simulink model "test_vehicle_model"  (R2016b)
settings: Solver=VariableStepAuto  StartTime=t_start  StopTime=t_stop  RelTol=1e-9  EnableMultiTasking=on
values from neighbouring files (symbols this model uses):
  a = 3.75    [test_vehicle.m]    (also in test_vehicle_model.m = 3.5)
  B = 5    [test_vehicle.m]    (also in test_vehicle_model.m)
  b = L - a    (= 3.25)    [test_vehicle.m]    (also in test_vehicle_model.m = 3.5)
  disturb_time = 5    [test_vehicle.m]
  disturb_val = 20    [test_vehicle.m]
  gear_ratio = 1/4.1    (= 0.243902439024)    [test_vehicle.m]    (also in test_vehicle_model.m = 1)
  I = 210000/(12^2)    (= 1458.33333333)    [test_vehicle.m]    (also in test_vehicle_model.m = 217852)
  input = [5000 50]    [test_vehicle.m]
  k_motor = 167    [test_vehicle.m]    (also in test_vehicle_model.m = 1)
  Ka = m*.15*180/(2*pi)    (= 40.0358707778)    [test_vehicle.m]    (also in test_vehicle_model.m = 0.5)
  Kx = m*.15*180/(2*pi)    (= 40.0358707778)    [test_vehicle.m]    (also in test_vehicle_model.m = 0.5)
  m = 300/32.2    (= 9.31677018634)    [test_vehicle.m]    (also in test_vehicle_model.m = 150)
  R = 4/12    (= 0.333333333333)    [test_vehicle.m]
  speed_D = 0    [test_vehicle.m]
  speed_I = 0    [test_vehicle.m]
  speed_N = 100    [test_vehicle.m]
  speed_P = 100    [test_vehicle.m]
  speed_sp = 30    [test_vehicle.m]
  steer_D = 0.1    [test_vehicle.m]
  steer_I = 0    [test_vehicle.m]
  steer_N = 1000    [test_vehicle.m]
  steer_P = 10    [test_vehicle.m]
  t_motor = 0.025    [test_vehicle.m]    (also in test_vehicle_model.m = 1)
  u_start = 0.01    [test_vehicle.m]
libraries: simulink x2
settings Model: Creator=jbarr  LastModifiedBy=john
settings SolverCC: ZeroCrossAlgorithm=Adaptive
settings OptimizationCC: LifeSpan=1
settings DebuggingCC: SFExecutionAtInitializationDiag=none

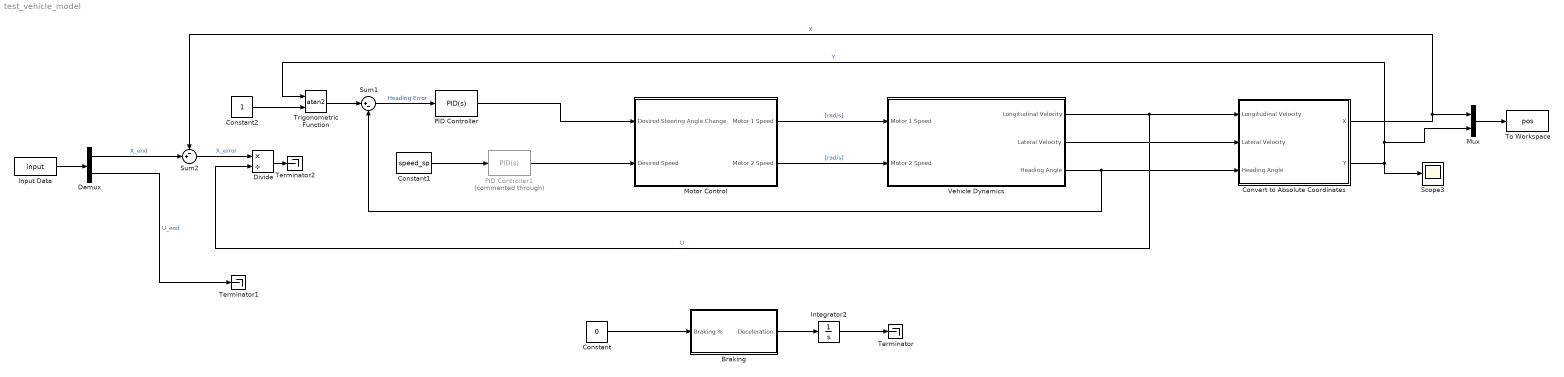
== system test_vehicle_model ==
  "Braking " : Subsystem
  Constant : Constant  Value=0
  Constant1 : Constant  Value=speed_sp
  Constant2 : Constant
  Convert to Absolute Coordinates : Subsystem
  Demux : Demux  Outputs=2
  Divide : Product  Inputs=*/
  Input Data : Constant  Value=input
  Integrator2 : Integrator  InitialCondition=0.001
  "Motor Control " : Subsystem
  Mux : Mux  Inputs=2
  PID Controller : simulink/Continuous/PID Controller  Controller=PID  TimeDomain=Continuous-time  SampleTime=-1  IntegratorMethod=Forward Euler  FilterMethod=Forward Euler  Form=Ideal  UseFilter=on  ControllerParametersSource=internal  P=steer_P  I=steer_I  D=steer_D  N=steer_N  InitialConditionSource=internal  InitialConditionForIntegrator=0  InitialConditionForFilter=0  ExternalReset=none  LimitOutput=off  UpperSaturationLimit=100  LowerSaturationLimit=0  LinearizeAsGain=on  AntiWindupMode=none  Kb=1  TrackingMode=off  Kt=1  PParamMin=[]  PParamMax=[]  IParamMin=[]  IParamMax=[]  DParamMin=[]  DParamMax=[]  NParamMin=[]  NParamMax=[]  KbParamMin=[]  KbParamMax=[]  KtParamMin=[]  KtParamMax=[]  POutMin=[]  POutMax=[]  IOutMin=[]  IOutMax=[]  DOutMin=[]  DOutMax=[]  NOutMin=[]  NOutMax=[]  KbOutMin=[]  KbOutMax=[]  KtOutMin=[]  KtOutMax=[]  IntegratorOutMin=[]  IntegratorOutMax=[]  FilterOutMin=[]  FilterOutMax=[]  SumOutMin=[]  SumOutMax=[]  SumI1OutMin=[]  SumI1OutMax=[]  SumI2OutMin=[]  SumI2OutMax=[]  SumI3OutMin=[]  SumI3OutMax=[]  SumDOutMin=[]  SumDOutMax=[]  SaturationOutMin=[]  SaturationOutMax=[]  IntegratorContinuousStateAttributes=''  IntegratorStateMustResolveToSignalObject=off  IntegratorRTWStateStorageClass=Auto  FilterContinuousStateAttributes=''  FilterStateMustResolveToSignalObject=off  FilterRTWStateStorageClass=Auto  DifferentiatorICPrevScaledInput=0  DifferentiatorOutMin=[]  DifferentiatorOutMax=[]
  PID Controller1 : simulink/Continuous/PID Controller  Commented=through  Controller=PID  TimeDomain=Continuous-time  SampleTime=-1  IntegratorMethod=Forward Euler  FilterMethod=Forward Euler  Form=Ideal  UseFilter=on  ControllerParametersSource=internal  P=speed_P  I=speed_I  D=speed_D  N=speed_N  InitialConditionSource=internal  InitialConditionForIntegrator=0  InitialConditionForFilter=0  ExternalReset=none  LimitOutput=off  UpperSaturationLimit=100  LowerSaturationLimit=0  LinearizeAsGain=on  AntiWindupMode=none  Kb=1  TrackingMode=off  Kt=1  PParamMin=[]  PParamMax=[]  IParamMin=[]  IParamMax=[]  DParamMin=[]  DParamMax=[]  NParamMin=[]  NParamMax=[]  KbParamMin=[]  KbParamMax=[]  KtParamMin=[]  KtParamMax=[]  POutMin=[]  POutMax=[]  IOutMin=[]  IOutMax=[]  DOutMin=[]  DOutMax=[]  NOutMin=[]  NOutMax=[]  KbOutMin=[]  KbOutMax=[]  KtOutMin=[]  KtOutMax=[]  IntegratorOutMin=[]  IntegratorOutMax=[]  FilterOutMin=[]  FilterOutMax=[]  SumOutMin=[]  SumOutMax=[]  SumI1OutMin=[]  SumI1OutMax=[]  SumI2OutMin=[]  SumI2OutMax=[]  SumI3OutMin=[]  SumI3OutMax=[]  SumDOutMin=[]  SumDOutMax=[]  SaturationOutMin=[]  SaturationOutMax=[]  IntegratorContinuousStateAttributes=''  IntegratorStateMustResolveToSignalObject=off  IntegratorRTWStateStorageClass=Auto  FilterContinuousStateAttributes=''  FilterStateMustResolveToSignalObject=off  FilterRTWStateStorageClass=Auto  DifferentiatorICPrevScaledInput=0  DifferentiatorOutMin=[]  DifferentiatorOutMax=[]
  Scope3 : Scope
  Sum1 : Sum  Inputs=|+-
  Sum2 : Sum  Inputs=-+|
  Terminator : Terminator
  Terminator1 : Terminator
  Terminator2 : Terminator
  To Workspace : ToWorkspace  VariableName=pos  SampleTime=-1
  Trigonometric Function : Trigonometry  Operator=atan2
  Vehicle Dynamics : Subsystem
  wires:
  "Motor Control "/1(Motor 1 Speed) -> Vehicle Dynamics/1(Motor 1 Speed)  "[rad/s]"
  Mux/1 -> To Workspace/1
  Convert to Absolute Coordinates/2(Y) -> Scope3/1, Trigonometric Function/1, Mux/2  "Y"
  Convert to Absolute Coordinates/1(X) -> Sum2/1, Mux/1  "X"
  "Braking "/1(Deceleration) -> Integrator2/1
  Vehicle Dynamics/1(Longitudinal Velocity) -> Divide/2, Convert to Absolute Coordinates/1(Longitudinal Velocity)  "U"
  Constant/1 -> "Braking "/1(Braking %)
  Sum1/1 -> PID Controller/1  "Heading Error"
  "Motor Control "/2(Motor 2 Speed) -> Vehicle Dynamics/2(Motor 2 Speed)  "[rad/s]"
  PID Controller/1 -> "Motor Control "/1(Desired Steering Angle Change)
  PID Controller1/1 -> "Motor Control "/2(Desired Speed)
  Integrator2/1 -> Terminator/1
  Vehicle Dynamics/2(Lateral Velocity) -> Convert to Absolute Coordinates/2(Lateral Velocity)
  Input Data/1 -> Demux/1
  Demux/1 -> Sum2/2  "X_end"
  Sum2/1 -> Divide/1  "X_error"
  Demux/2 -> Terminator1/1  "U_end"
  Trigonometric Function/1 -> Sum1/1
  Constant1/1 -> PID Controller1/1
  Divide/1 -> Terminator2/1
  Vehicle Dynamics/3(Heading Angle) -> Sum1/2, Convert to Absolute Coordinates/3(Heading Angle)
  Constant2/1 -> Trigonometric Function/2

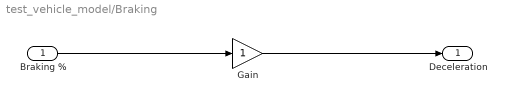
== system test_vehicle_model/Braking  ==
  Braking % : Inport
  Gain : Gain
  Deceleration : Outport
  wires:
  Gain/1 -> Deceleration/1
  Braking %/1 -> Gain/1

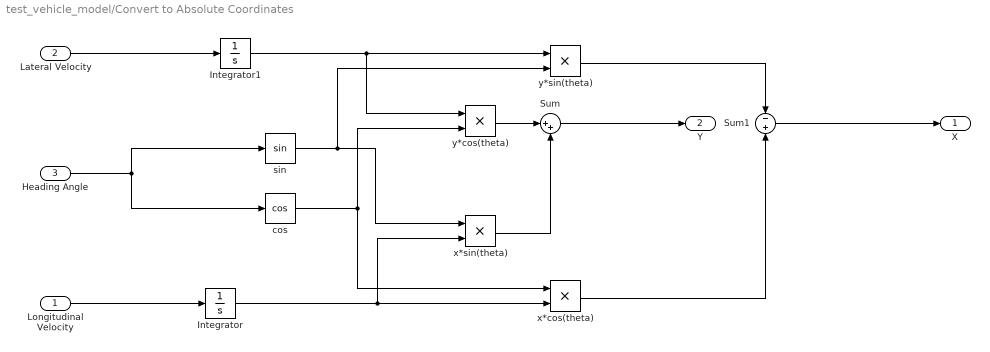
== system test_vehicle_model/Convert to Absolute Coordinates ==
  Longitudinal Velocity : Inport
  Lateral Velocity : Inport  Port=2
  Heading Angle : Inport  Port=3
  Integrator : Integrator  InitialCondition=0.001
  Integrator1 : Integrator
  Sum : Sum  Inputs=|++
  Sum1 : Sum  Inputs=-+
  cos : Trigonometry  Operator=cos
  sin : Trigonometry
  x*cos(theta) : Product
  x*sin(theta) : Product
  y*cos(theta) : Product
  y*sin(theta) : Product
  X : Outport
  Y : Outport  Port=2
  wires:
  Longitudinal Velocity/1 -> Integrator/1
  cos/1 -> y*cos(theta)/2, x*cos(theta)/1
  sin/1 -> x*sin(theta)/1, y*sin(theta)/2
  x*cos(theta)/1 -> Sum1/2
  x*sin(theta)/1 -> Sum/2
  y*cos(theta)/1 -> Sum/1
  y*sin(theta)/1 -> Sum1/1
  Integrator1/1 -> y*cos(theta)/1, y*sin(theta)/1
  Integrator/1 -> x*sin(theta)/2, x*cos(theta)/2
  Heading Angle/1 -> sin/1, cos/1
  Sum1/1 -> X/1
  Lateral Velocity/1 -> Integrator1/1
  Sum/1 -> Y/1

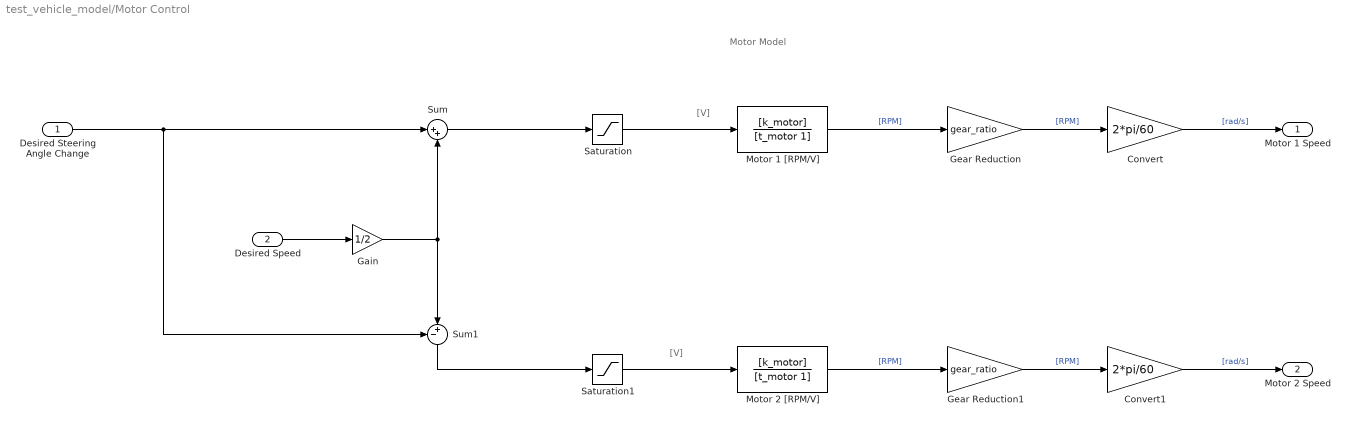
== system test_vehicle_model/Motor Control  ==
  note: [V]
  note: Motor Model
  note: [V]
  Desired Steering Angle Change : Inport
  Desired Speed : Inport  Port=2
  Convert : Gain  Gain=2*pi/60
  Convert1 : Gain  Gain=2*pi/60
  Gain : Gain  Gain=1/2
  Gear Reduction : Gain  Gain=gear_ratio
  Gear Reduction1 : Gain  Gain=gear_ratio
  "Motor 1 [RPM/V] " : TransferFcn  Numerator=[k_motor]  Denominator=[t_motor 1]
  Motor 2 [RPM/V] : TransferFcn  Numerator=[k_motor]  Denominator=[t_motor 1]
  Saturation : Saturate  UpperLimit=36  LowerLimit=-36
  Saturation1 : Saturate  UpperLimit=36  LowerLimit=-36
  Sum : Sum  Inputs=|++
  Sum1 : Sum  Inputs=-+|
  Motor 1 Speed : Outport
  Motor 2 Speed : Outport  Port=2
  wires:
  "Motor 1 [RPM/V] "/1 -> Gear Reduction/1  "[RPM]"
  Gear Reduction/1 -> Convert/1  "[RPM]"
  Convert/1 -> Motor 1 Speed/1  "[rad/s]"
  Saturation/1 -> "Motor 1 [RPM/V] "/1
  Motor 2 [RPM/V]/1 -> Gear Reduction1/1  "[RPM]"
  Gear Reduction1/1 -> Convert1/1  "[RPM]"
  Convert1/1 -> Motor 2 Speed/1  "[rad/s]"
  Saturation1/1 -> Motor 2 [RPM/V]/1
  Desired Steering Angle Change/1 -> Sum/1, Sum1/1
  Sum/1 -> Saturation/1
  Sum1/1 -> Saturation1/1
  Desired Speed/1 -> Gain/1
  Gain/1 -> Sum1/2, Sum/2

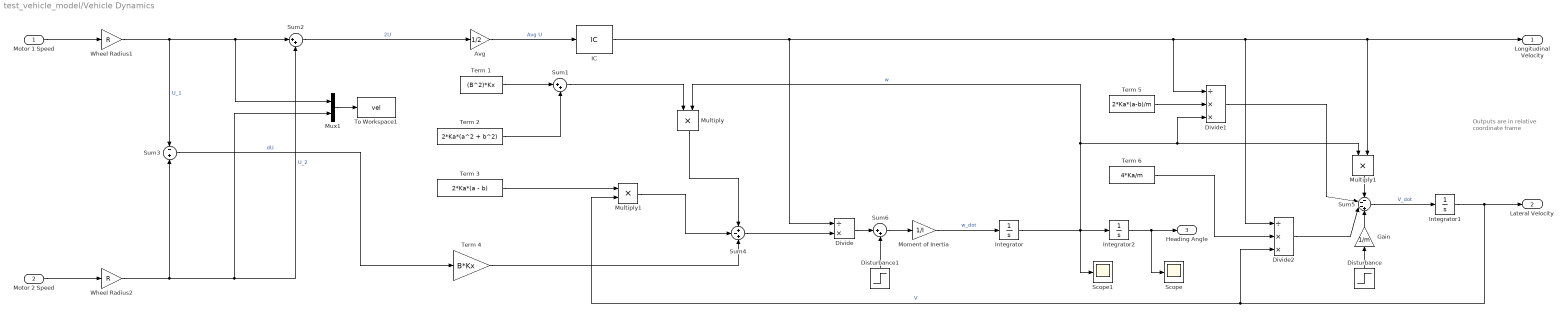
== system test_vehicle_model/Vehicle Dynamics ==
  note: Outputs are in relative
      | coordinate frame
  Motor 1 Speed : Inport
  Motor 2 Speed : Inport  Port=2
  Avg : Gain  Gain=1/2
  Disturbance : Step  Time=disturb_time  After=disturb_val  SampleTime=0
  Disturbance1 : Step  Time=disturb_time  After=disturb_val  SampleTime=0
  Divide : Product  Inputs=/*
  Divide1 : Product  Inputs=/**
  Divide2 : Product  Inputs=/**
  Gain : Gain  Gain=1/m
  IC : InitialCondition  Value=u_start
  Integrator : Integrator
  Integrator1 : Integrator
  Integrator2 : Integrator
  Moment of Inertia : Gain  Gain=1/I
  Multiply : Product  Inputs=**
  Multiply1 : Product  Inputs=**
  "Multiply1\t" : Product  Inputs=**
  Mux1 : Mux  Inputs=2
  Scope : Scope
  Scope1 : Scope
  Sum1 : Sum  Inputs=|++
  Sum2 : Sum  Inputs=|++
  Sum3 : Sum  Inputs=-+
  Sum4 : Sum  Inputs=+-+
  Sum5 : Sum  Inputs=---+
  Sum6 : Sum  Inputs=|++
  Term 1 : Constant  Value=(B^2)*Kx
  Term 2 : Constant  Value=2*Ka*(a^2 + b^2)
  Term 3 : Constant  Value=2*Ka*(a - b)
  Term 4 : Gain  Gain=B*Kx
  Term 5 : Constant  Value=2*Ka*(a-b)/m
  Term 6 : Constant  Value=4*Ka/m
  To Workspace1 : ToWorkspace  VariableName=vel  SampleTime=-1
  Wheel Radius1 : Gain  Gain=R
  Wheel Radius2 : Gain  Gain=R
  Longitudinal Velocity : Outport
  Lateral Velocity : Outport  Port=2
  Heading Angle : Outport  Port=3
  wires:
  Motor 1 Speed/1 -> Wheel Radius1/1
  Motor 2 Speed/1 -> Wheel Radius2/1
  Wheel Radius1/1 -> Sum2/1, Mux1/1, Sum3/1  "U_1"
  Wheel Radius2/1 -> Sum2/2, Mux1/2, Sum3/2  "U_2"
  Sum2/1 -> Avg/1  "2U"
  Avg/1 -> IC/1  "Avg U"
  Sum3/1 -> Term 4/1  "dU"
  Integrator/1 -> Scope1/1, Multiply/2, Divide1/3, "Multiply1\t"/1, Integrator2/1  "w"
  Moment of Inertia/1 -> Integrator/1  "w_dot"
  Integrator1/1 -> Lateral Velocity/1, Divide2/3, Multiply1/2  "V"
  Term 2/1 -> Sum1/2
  Term 1/1 -> Sum1/1
  Sum1/1 -> Multiply/1
  Term 3/1 -> Multiply1/1
  Sum4/1 -> Divide/2
  Term 4/1 -> Sum4/3
  Multiply1/1 -> Sum4/2
  Multiply/1 -> Sum4/1
  Term 5/1 -> Divide1/2
  Term 6/1 -> Divide2/2
  Divide1/1 -> Sum5/2
  Divide2/1 -> Sum5/3
  "Multiply1\t"/1 -> Sum5/1
  Sum5/1 -> Integrator1/1  "V_dot"
  IC/1 -> Divide/1, Divide2/1, "Multiply1\t"/2, Longitudinal Velocity/1, Divide1/1
  Integrator2/1 -> Scope/1, Heading Angle/1
  Disturbance/1 -> Gain/1
  Gain/1 -> Sum5/4
  Divide/1 -> Sum6/1
  Sum6/1 -> Moment of Inertia/1
  Disturbance1/1 -> Sum6/2
  Mux1/1 -> To Workspace1/1
